simulink model "HW1_Q2"  (R2018a)
settings: Solver=VariableStepAuto  StartTime=0.0  StopTime=50  RelTol=1e-3
settings Model: Creator=Halil Temurtaş  LastModifiedBy=Halil Temurtaş

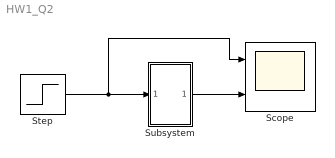
== system HW1_Q2 ==
  Scope : Scope  NumInputPorts=2
  Step : Step  Time=0  After=14  SampleTime=0
  Subsystem : Subsystem
  wires:
  Step/1 -> Scope/1, Subsystem/1(In1)
  Subsystem/1(Out1) -> Scope/2

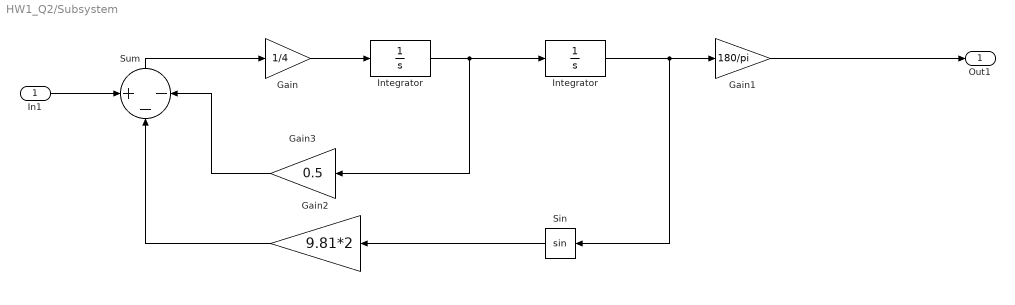
== system HW1_Q2/Subsystem ==
  In1 : Inport
  Gain : Gain  Gain=1/4
  Gain1 : Gain  Gain=180/pi
  Gain2 : Gain  Gain=9.81*2
  Gain3 : Gain  Gain=0.5
  Integrator : TransferFcn  Denominator=[1 0]
  "Integrator " : TransferFcn  Denominator=[1 0]
  Sin : Trigonometry
  Sum : Sum  Inputs=+--
  Out1 : Outport
  wires:
  "Integrator "/1 -> Sin/1, Gain1/1
  Integrator/1 -> Gain3/1, "Integrator "/1
  Gain1/1 -> Out1/1
  Sum/1 -> Gain/1
  Gain3/1 -> Sum/3
  Gain/1 -> Integrator/1
  Gain2/1 -> Sum/2
  Sin/1 -> Gain2/1
  In1/1 -> Sum/1
